simulink model "orion_casestudy_1"  (R2023a)
settings: Solver=VariableStepAuto  StartTime=0.0  StopTime=30  RelTol=1e-3
InitFcn:
  | RandStream.setGlobalStream(RandStream('mt19937ar','seed',sum(100*clock)));
undefined symbols (not defined in the file or in its folder): m, n
settings Model: Creator=simon  LastModifiedBy=simon
settings OptimizationCC: AccelVerboseBuild=on
settings DebuggingCC: UnderSpecifiedDataTypeMsg=warning  UnderSpecifiedDimensionMsg=warning

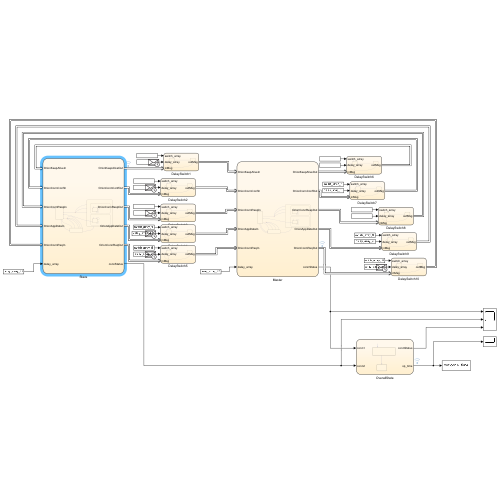
[thumbnail: Simulink's stored preview of the top-level diagram]
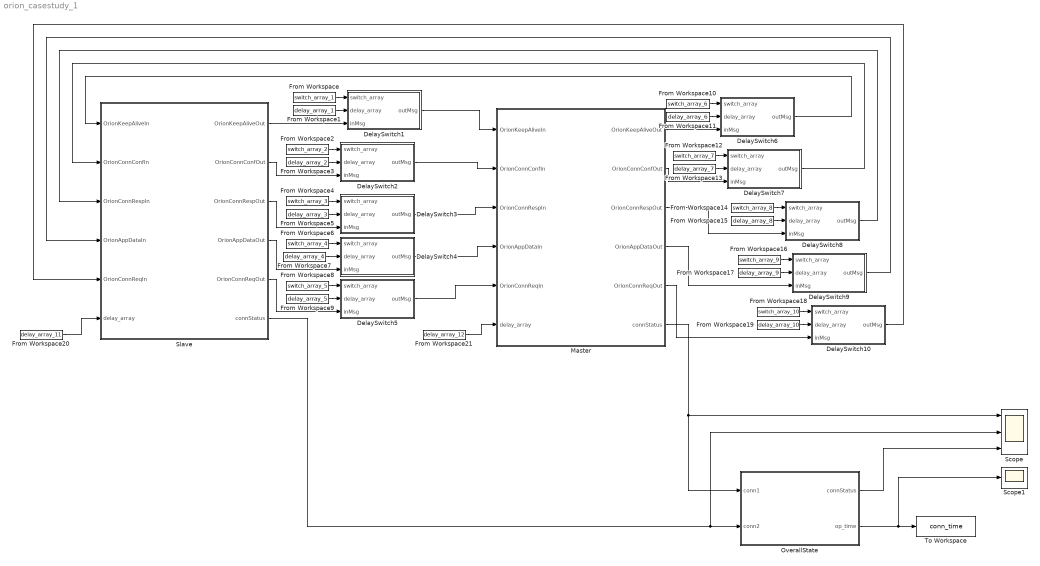
== system orion_casestudy_1 ==
  DelaySwitch1 : Stateflow chart  TreatAsAtomicUnit=on
  DelaySwitch10 : Stateflow chart  TreatAsAtomicUnit=on
  DelaySwitch2 : Stateflow chart  TreatAsAtomicUnit=on
  DelaySwitch3 : Stateflow chart  TreatAsAtomicUnit=on
  DelaySwitch4 : Stateflow chart  TreatAsAtomicUnit=on
  DelaySwitch5 : Stateflow chart  TreatAsAtomicUnit=on
  DelaySwitch6 : Stateflow chart  TreatAsAtomicUnit=on
  DelaySwitch7 : Stateflow chart  TreatAsAtomicUnit=on
  DelaySwitch8 : Stateflow chart  TreatAsAtomicUnit=on
  DelaySwitch9 : Stateflow chart  TreatAsAtomicUnit=on
  From Workspace : FromWorkspace  VariableName=switch_array_1  SampleTime=-1  Interpolate=off  ZeroCross=off  OutputAfterFinalValue=Holding final value
  From Workspace1 : FromWorkspace  VariableName=delay_array_1  SampleTime=-1  Interpolate=off  ZeroCross=off  OutputAfterFinalValue=Holding final value
  From Workspace10 : FromWorkspace  VariableName=switch_array_6  SampleTime=-1  Interpolate=off  ZeroCross=off  OutputAfterFinalValue=Holding final value
  From Workspace11 : FromWorkspace  VariableName=delay_array_6  SampleTime=-1  Interpolate=off  ZeroCross=off  OutputAfterFinalValue=Holding final value
  From Workspace12 : FromWorkspace  VariableName=switch_array_7  SampleTime=-1  Interpolate=off  ZeroCross=off  OutputAfterFinalValue=Holding final value
  From Workspace13 : FromWorkspace  VariableName=delay_array_7  SampleTime=-1  Interpolate=off  ZeroCross=off  OutputAfterFinalValue=Holding final value
  From Workspace14 : FromWorkspace  VariableName=switch_array_8  SampleTime=-1  Interpolate=off  ZeroCross=off  OutputAfterFinalValue=Holding final value
  From Workspace15 : FromWorkspace  VariableName=delay_array_8  SampleTime=-1  Interpolate=off  ZeroCross=off  OutputAfterFinalValue=Holding final value
  From Workspace16 : FromWorkspace  VariableName=switch_array_9  SampleTime=-1  Interpolate=off  ZeroCross=off  OutputAfterFinalValue=Holding final value
  From Workspace17 : FromWorkspace  VariableName=delay_array_9  SampleTime=-1  Interpolate=off  ZeroCross=off  OutputAfterFinalValue=Holding final value
  From Workspace18 : FromWorkspace  VariableName=switch_array_10  SampleTime=-1  Interpolate=off  ZeroCross=off  OutputAfterFinalValue=Holding final value
  From Workspace19 : FromWorkspace  VariableName=delay_array_10  SampleTime=-1  Interpolate=off  ZeroCross=off  OutputAfterFinalValue=Holding final value
  From Workspace2 : FromWorkspace  VariableName=switch_array_2  SampleTime=-1  Interpolate=off  ZeroCross=off  OutputAfterFinalValue=Holding final value
  From Workspace20 : FromWorkspace  VariableName=delay_array_11  SampleTime=-1  Interpolate=off  ZeroCross=off  OutputAfterFinalValue=Holding final value
  From Workspace21 : FromWorkspace  VariableName=delay_array_12  SampleTime=-1  Interpolate=off  ZeroCross=off  OutputAfterFinalValue=Holding final value
  From Workspace3 : FromWorkspace  VariableName=delay_array_2  SampleTime=-1  Interpolate=off  ZeroCross=off  OutputAfterFinalValue=Holding final value
  From Workspace4 : FromWorkspace  VariableName=switch_array_3  SampleTime=-1  Interpolate=off  ZeroCross=off  OutputAfterFinalValue=Holding final value
  From Workspace5 : FromWorkspace  VariableName=delay_array_3  SampleTime=-1  Interpolate=off  ZeroCross=off  OutputAfterFinalValue=Holding final value
  From Workspace6 : FromWorkspace  VariableName=switch_array_4  SampleTime=-1  Interpolate=off  ZeroCross=off  OutputAfterFinalValue=Holding final value
  From Workspace7 : FromWorkspace  VariableName=delay_array_4  SampleTime=-1  Interpolate=off  ZeroCross=off  OutputAfterFinalValue=Holding final value
  From Workspace8 : FromWorkspace  VariableName=switch_array_5  SampleTime=-1  Interpolate=off  ZeroCross=off  OutputAfterFinalValue=Holding final value
  From Workspace9 : FromWorkspace  VariableName=delay_array_5  SampleTime=-1  Interpolate=off  ZeroCross=off  OutputAfterFinalValue=Holding final value
  Master : Stateflow chart  TreatAsAtomicUnit=on
      settings: PortSchema="{\"entries\":[{\"content\":{\"sides\":[{\"content\":{\"connectorIds\":[\"In2\",\"In3\",\"In5\",\"In4\",\"In6\",\"In1\"]},\"type\":\"ConnectorPlacement.EquallySpacedRectSide\",\"uuid\":\"93190a42-59cb-4d31-aa72-080cef5549db\"},{\"content\":{\"connectorIds\":[\"Out1\",\"Out2\",\"Out3\",\"Out4\",\"Out5\",\"Out6\"],\"side\":\"RIGHT\"},\"type\":\"ConnectorPlacement.EquallySpacedRectSide\",\"uuid\":\"4a04e977-42e8-4d3e-8e66-86884aeb71d4\"},{\"content\":{\"side\":\"TOP\"},\"type\":\"ConnectorPlacement.EquallySpacedRectSide\",\"uuid\":\"cb7bc3bf-3799-42a3-9f12-c8b4e7be85f7\"},{\"content\":{\"side\":\"BOTTOM\"},\"type\":\"ConnectorPlacement.EquallySpacedRectSide\",\"uuid\":\"934a78a5-af7b-46d0-ad43-c65a76addb63\"}]},\"type\":\"ConnectorPlacement.EquallySpacedConnector\",\"uuid\":\"bab253c4-7746-42e8-9b4d-6fa7ff1cc3b1\"}],\"packageUris\":[\"http://schema.mathworks.com/mf0/Connector/R2020b\"],\"version\":\"1.0\"}"
  OverallState : Stateflow chart  TreatAsAtomicUnit=on
  Scope : Scope  NumInputPorts=3
  Scope1 : Scope
  Slave : Stateflow chart  TreatAsAtomicUnit=on
      settings: PortSchema="{\"entries\":[{\"content\":{\"sides\":[{\"content\":{\"connectorIds\":[\"In1\",\"In5\",\"In3\",\"In2\",\"In4\",\"In6\"]},\"type\":\"ConnectorPlacement.EquallySpacedRectSide\",\"uuid\":\"93190a42-59cb-4d31-aa72-080cef5549db\"},{\"content\":{\"connectorIds\":[\"Out3\",\"Out1\",\"Out2\",\"Out4\",\"Out5\",\"Out6\"],\"side\":\"RIGHT\"},\"type\":\"ConnectorPlacement.EquallySpacedRectSide\",\"uuid\":\"4a04e977-42e8-4d3e-8e66-86884aeb71d4\"},{\"content\":{\"side\":\"TOP\"},\"type\":\"ConnectorPlacement.EquallySpacedRectSide\",\"uuid\":\"cb7bc3bf-3799-42a3-9f12-c8b4e7be85f7\"}]},\"type\":\"ConnectorPlacement.EquallySpacedConnector\",\"uuid\":\"bab253c4-7746-42e8-9b4d-6fa7ff1cc3b1\"}],\"packageUris\":[\"http://schema.mathworks.com/mf0/Connector/R2020b\"],\"version\":\"1.0\"}"
  To Workspace : ToWorkspace  VariableName=conn_time  SaveFormat=Timeseries  SampleTime=-1
  wires:
  Slave/4(OrionAppDataOut) -> DelaySwitch4/3(inMsg)
  Slave/2(OrionConnRespOut) -> DelaySwitch3/3(inMsg)
  Slave/1(OrionConnConfOut) -> DelaySwitch2/3(inMsg)
  Slave/3(OrionKeepAliveOut) -> DelaySwitch1/3(inMsg)
  DelaySwitch3/1(outMsg) -> Master/5(OrionConnRespIn)
  DelaySwitch4/1(outMsg) -> Master/4(OrionAppDataIn)
  DelaySwitch2/1(outMsg) -> Master/3(OrionConnConfIn)
  DelaySwitch1/1(outMsg) -> Master/2(OrionKeepAliveIn)
  DelaySwitch10/1(outMsg) -> Slave/4(OrionConnReqIn)
  DelaySwitch9/1(outMsg) -> Slave/2(OrionAppDataIn)
  DelaySwitch8/1(outMsg) -> Slave/3(OrionConnRespIn)
  DelaySwitch7/1(outMsg) -> Slave/5(OrionConnConfIn)
  DelaySwitch6/1(outMsg) -> Slave/1(OrionKeepAliveIn)
  Master/6(connStatus) -> OverallState/1(conn1), Scope/1
  Slave/6(connStatus) -> Scope/2, OverallState/2(conn2)
  OverallState/1(connStatus) -> Scope/3
  OverallState/2(op_time) -> Scope1/1, To Workspace/1
  From Workspace/1 -> DelaySwitch1/1(switch_array)
  From Workspace1/1 -> DelaySwitch1/2(delay_array)
  From Workspace3/1 -> DelaySwitch2/2(delay_array)
  From Workspace2/1 -> DelaySwitch2/1(switch_array)
  From Workspace4/1 -> DelaySwitch3/1(switch_array)
  From Workspace5/1 -> DelaySwitch3/2(delay_array)
  From Workspace7/1 -> DelaySwitch4/2(delay_array)
  From Workspace6/1 -> DelaySwitch4/1(switch_array)
  From Workspace8/1 -> DelaySwitch5/1(switch_array)
  From Workspace9/1 -> DelaySwitch5/2(delay_array)
  Slave/5(OrionConnReqOut) -> DelaySwitch5/3(inMsg)
  DelaySwitch5/1(outMsg) -> Master/6(OrionConnReqIn)
  From Workspace11/1 -> DelaySwitch6/2(delay_array)
  From Workspace10/1 -> DelaySwitch6/1(switch_array)
  Master/1(OrionKeepAliveOut) -> DelaySwitch6/3(inMsg)
  From Workspace12/1 -> DelaySwitch7/1(switch_array)
  From Workspace13/1 -> DelaySwitch7/2(delay_array)
  From Workspace15/1 -> DelaySwitch8/2(delay_array)
  From Workspace14/1 -> DelaySwitch8/1(switch_array)
  Master/2(OrionConnConfOut) -> DelaySwitch7/3(inMsg)
  Master/3(OrionConnRespOut) -> DelaySwitch8/3(inMsg)
  From Workspace16/1 -> DelaySwitch9/1(switch_array)
  From Workspace17/1 -> DelaySwitch9/2(delay_array)
  From Workspace19/1 -> DelaySwitch10/2(delay_array)
  From Workspace18/1 -> DelaySwitch10/1(switch_array)
  Master/4(OrionAppDataOut) -> DelaySwitch9/3(inMsg)
  Master/5(OrionConnReqOut) -> DelaySwitch10/3(inMsg)
  From Workspace20/1 -> Slave/6(delay_array)
  From Workspace21/1 -> Master/1(delay_array)

== stateflow chart orion_casestudy_1/DelaySwitch3 ==
  state Operation
  state Sending
  (default) -> Operation : {i=0;}
  (junction 7) -> Operation [order 2]
  Sending -> Operation : after(delay_array(i),msec)
      | {receive(inMsg);outMsg.data=0;send(outMsg);}
  Operation -> (junction 7) : inMsg{i = i + 1;}
  (junction 7) -> Sending [order 1] : [switch_array(i)==0]
  data: switch_array input; delay_array input; outMsg output; inMsg input; i local

== stateflow chart orion_casestudy_1/DelaySwitch4 ==
  state Operation
  state Sending
  (default) -> Operation : {i=0;}
  (junction 7) -> Operation [order 2]
  Sending -> Operation : after(delay_array(i),msec)
      | {receive(inMsg);outMsg.data=0;send(outMsg);}
  Operation -> (junction 7) : inMsg{i = i + 1;}
  (junction 7) -> Sending [order 1] : [switch_array(i)==0]
  data: switch_array input; delay_array input; outMsg output; inMsg input; i local

== stateflow chart orion_casestudy_1/DelaySwitch5 ==
  state Operation
  state Sending
  (default) -> Operation : {i=0;}
  (junction 7) -> Operation [order 2]
  Sending -> Operation : after(delay_array(i),msec)
      | {receive(inMsg);outMsg.data=0;send(outMsg);}
  Operation -> (junction 7) : inMsg{i = i + 1;}
  (junction 7) -> Sending [order 1] : [switch_array(i)==0]
  data: switch_array input; delay_array input; outMsg output; inMsg input; i local

== stateflow chart orion_casestudy_1/DelaySwitch6 ==
  state Operation
  state Sending
  (default) -> Operation : {i=0;}
  (junction 7) -> Operation [order 2]
  Sending -> Operation : after(delay_array(i),msec)
      | {receive(inMsg);outMsg.data=0;send(outMsg);}
  Operation -> (junction 7) : inMsg{i = i + 1;}
  (junction 7) -> Sending [order 1] : [switch_array(i)==0]
  data: switch_array input; delay_array input; outMsg output; inMsg input; i local

== stateflow chart orion_casestudy_1/Slave ==
  settings: updateMethod=CONTINUOUS
  state Connected
    entry:
    connStatus=2;
    state KeepAliveSendTimeout [parallel]
      settings: executionOrder=1
      state KeepAliveSend
      (default) -> KeepAliveSend
      KeepAliveSend -> KeepAliveSend [order 1] : after(delay_array(i)*5,msec)
          |  {OrionKeepAliveOut.data=0;
          | send(OrionKeepAliveOut);i = i + 1;}
      KeepAliveSend -> KeepAliveSend [order 2] : SendDataIn
          | {OrionAppDataOut.data=0;
          | send(OrionAppDataOut);}
    state KeepAliveRecieveTimeout [parallel]
      settings: executionOrder=2
      state KeepAlineRec
      (default) -> KeepAlineRec
      KeepAlineRec -> KeepAlineRec [order 2] : OrionKeepAliveIn
      KeepAlineRec -> KeepAlineRec [order 3] : OrionAppDataIn
  state Closed
    entry:
    connStatus=0;
  state Connecting
    entry:
    connStatus=1;
  Connected -> (junction 6) [order 2] : OrionConnRespIn
  Connected -> (junction 6) [order 3] : OrionConnReqIn
  (default) -> Closed : {i=1;}
  (junction 6) -> Closed
  Connected -> (junction 6) [order 1] : OrionConnConfIn
  KeepAlineRec -> Closed [order 1] : after(delay_array(i)*5,msec)
      | {i = i + 1;}
  Connecting -> (junction 36) [order 6] : OrionAppDataIn
  Connecting -> (junction 36) [order 5] : OrionConnReqIn
  (junction 36) -> Closed
  Connecting -> (junction 36) [order 4] : OrionConnRespIn
  Connecting -> (junction 36) [order 3] : OrionKeepAliveIn
  Closed -> Connecting : OrionConnReqIn
      | {OrionConnRespOut.data=0;
      | send(OrionConnRespOut);}
  Connecting -> Closed [order 1] : after(delay_array(i)*5,msec)
      | {i = i + 1;}
  Connecting -> Connected [order 2] : OrionConnConfIn{OrionConnConfOut.data=0;send(OrionConnConfOut);}
  data: OrionKeepAliveIn input; OrionConnConfOut output; OrionConnRespOut output; OrionKeepAliveOut output; OrionAppDataOut output; OrionAppDataIn input; OrionConnRespIn input; OrionConnReqIn input; OrionConnReqOut output size=1; connStatus output; SendDataIn local; OrionConnConfIn input; delay_array input; i local

== stateflow chart orion_casestudy_1/DelaySwitch7 ==
  state Operation
  state Sending
  (default) -> Operation : {i=0;}
  (junction 7) -> Operation [order 2]
  Sending -> Operation : after(delay_array(i),msec)
      | {receive(inMsg);outMsg.data=0;send(outMsg);}
  Operation -> (junction 7) : inMsg{i = i + 1;}
  (junction 7) -> Sending [order 1] : [switch_array(i)==0]
  data: switch_array input; delay_array input; outMsg output; inMsg input; i local

== stateflow chart orion_casestudy_1/DelaySwitch8 ==
  state Operation
  state Sending
  (default) -> Operation : {i=0;}
  (junction 7) -> Operation [order 2]
  Sending -> Operation : after(delay_array(i),msec)
      | {receive(inMsg);outMsg.data=0;send(outMsg);}
  Operation -> (junction 7) : inMsg{i = i + 1;}
  (junction 7) -> Sending [order 1] : [switch_array(i)==0]
  data: switch_array input; delay_array input; outMsg output; inMsg input; i local

== stateflow chart orion_casestudy_1/DelaySwitch9 ==
  state Operation
  state Sending
  (default) -> Operation : {i=0;}
  (junction 7) -> Operation [order 2]
  Sending -> Operation : after(delay_array(i),msec)
      | {receive(inMsg);outMsg.data=0;send(outMsg);}
  Operation -> (junction 7) : inMsg{i = i + 1;}
  (junction 7) -> Sending [order 1] : [switch_array(i)==0]
  data: switch_array input; delay_array input; outMsg output; inMsg input; i local

== stateflow chart orion_casestudy_1/DelaySwitch10 ==
  state Operation
  state Sending
  (default) -> Operation : {i=0;}
  (junction 7) -> Operation [order 2]
  Sending -> Operation : after(delay_array(i),msec)
      | {receive(inMsg);outMsg.data=0;send(outMsg);}
  Operation -> (junction 7) : inMsg{i = i + 1;}
  (junction 7) -> Sending [order 1] : [switch_array(i)==0]
  data: switch_array input; delay_array input; outMsg output; inMsg input; i local

== stateflow chart orion_casestudy_1/OverallState ==
  settings: updateMethod=CONTINUOUS
  state NotConnected
    op_time=temporalCount(msec);
  state Connected
    entry:
    connStatus=1;
  (default) -> NotConnected : {connStatus=0;
      | op_time=0;}
  NotConnected -> Connected : [conn1==2 && conn2==2]
  data: conn1 input; conn2 input; connStatus output; op_time output

== stateflow chart orion_casestudy_1/DelaySwitch1 ==
  state Operation
  state Sending
  (default) -> Operation : {i=0;}
  (junction 7) -> Operation [order 2]
  Sending -> Operation : after(delay_array(i),msec)
      | {receive(inMsg);outMsg.data=0;send(outMsg);}
  Operation -> (junction 7) : inMsg{i = i + 1;}
  (junction 7) -> Sending [order 1] : [switch_array(i)==0]
  data: switch_array input; delay_array input; outMsg output; inMsg input; i local

== stateflow chart orion_casestudy_1/DelaySwitch2 ==
  state Operation
  state Sending
  (default) -> Operation : {i=0;}
  (junction 7) -> Operation [order 2]
  Sending -> Operation : after(delay_array(i),msec)
      | {receive(inMsg);outMsg.data=0;send(outMsg);}
  Operation -> (junction 7) : inMsg{i = i + 1;}
  (junction 7) -> Sending [order 1] : [switch_array(i)==0]
  data: switch_array input; delay_array input; outMsg output; inMsg input; i local

== stateflow chart orion_casestudy_1/Master ==
  settings: updateMethod=CONTINUOUS
  state Connected
    entry:
    connStatus=2;
    state KeepAliveSendTimeout [parallel]
      settings: executionOrder=1
      state KeepAliveSend
      (default) -> KeepAliveSend
      KeepAliveSend -> KeepAliveSend [order 1] : after(delay_array(i)*5,msec)
          | {OrionKeepAliveOut.data=0;
          | send(OrionKeepAliveOut);
          | i = i + 1;}
      KeepAliveSend -> KeepAliveSend [order 2] : SendDataIn
          | {OrionAppDataOut.data=0;
          | send(OrionAppDataOut);}
    state KeepAliveRecieveTimeout [parallel]
      settings: executionOrder=2
      state KeepAlineRec
      (default) -> KeepAlineRec
      KeepAlineRec -> KeepAlineRec [order 2] : OrionKeepAliveIn
      KeepAlineRec -> KeepAlineRec [order 3] : OrionAppDataIn
  state Closed
    entry:
    connStatus=0;
  state Connecting
    entry:
    connStatus=1;
  Connected -> (junction 6) [order 1] : OrionConnConfIn
  (default) -> Closed : {i=1;}
  Connected -> (junction 6) [order 2] : OrionConnRespIn
  Connected -> (junction 6) [order 3] : OrionConnReqIn
  (junction 6) -> Closed
  KeepAlineRec -> Closed [order 1] : after(delay_array(i)*5,msec)
      | {i = i + 1;}
  Connecting -> (junction 36) [order 5] : OrionConnReqIn
  (junction 36) -> Closed
  Connecting -> (junction 36) [order 4] : OrionConnRespIn
  Connecting -> (junction 36) [order 2] : OrionKeepAliveIn
  Connecting -> Closed [order 3] : after(delay_array(i)*5,msec)
      | {i = i + 1;}
  Closed -> Connecting [order 2] : after(delay_array(i)*5,msec)
      | {OrionConnReqOut.data=0;send(OrionConnReqOut);i = i + 1;}
  Closed -> Connecting [order 1] : OrionConnReqIn
      | {OrionConnRespOut.data=0;send(OrionConnRespOut);}
  Connecting -> Connected [order 1] : OrionConnRespIn
      | {OrionConnConfOut.data=0;
      | send(OrionConnConfOut);}
  data: delay_array input; OrionKeepAliveOut output; OrionKeepAliveIn input; OrionConnConfOut output; OrionConnConfIn input; OrionConnRespOut output; OrionAppDataOut output; OrionAppDataIn input; OrionConnRespIn input; OrionConnReqIn input; OrionConnReqOut output; connStatus output; SendDataIn local; i local
